simulink model "FCSMPCmono"  (R2022b)
settings: Solver=FixedStepAuto  StartTime=0.0  StopTime=5  FixedStep=Tsimu  RelTol=1e-3
undefined symbols (not defined in the file or in its folder): A, B, Izmax, Lo, Ro, Ts, Tsimu, Vdc1, Vdc2, Vgx_peak, w
libraries: spsSeriesRLCBranchLib x11, spsCurrentMeasurementLib x8, spsIGBTDiodeLib x6, slpidlib x6, simulink x4, dspstat3 x3, spsVoltageMeasurementLib x3, spsDCVoltageSourceLib x2, spsControlledVoltageSourceLib x1, spsPVArrayLib x1, spsTriangleGeneratorLib x1, spspowerguiLib x1
settings Model: Creator=hardw  LastModifiedBy=Salas Híbridas PC9
settings DebuggingCC: UnconnectedInputMsg=warning  UnconnectedOutputMsg=warning  UnconnectedLineMsg=warning
settings ModelReferenceCC: EnableRefExpFcnMdlSchedulingChecks=on
settings RTWCC: DLArmComputeVersion=19.05

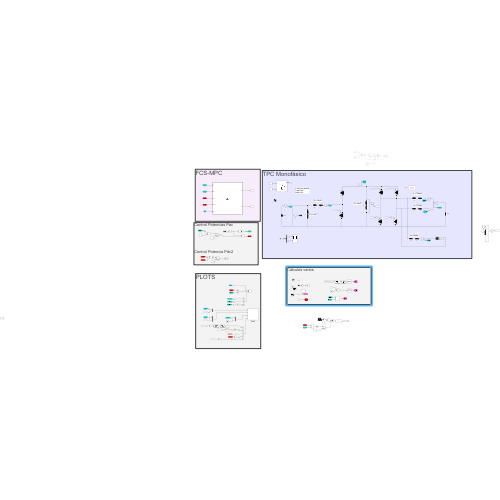
[thumbnail: Simulink's stored preview of the top-level diagram]
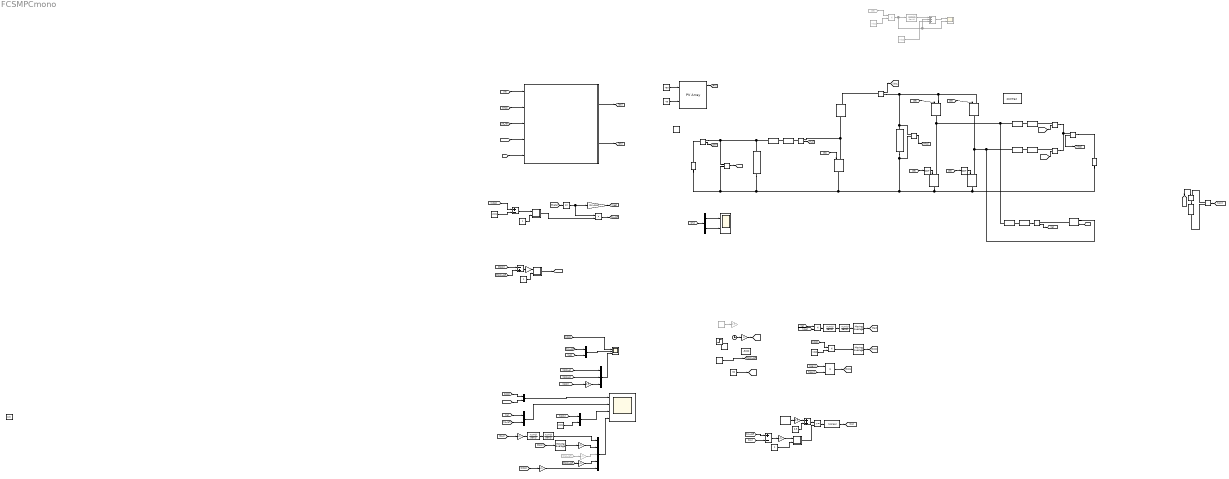
== system FCSMPCmono ==
  note: L=1mH
  note: 3 string en paralelo
      | Vmpp=42V
      | Impp=13A
  note: TPC Monofásico
  note: FCS-MPC
  note: PLOTS
  note: Control Potencias Pac
      |
      |
      |
      |
      |
      | Control Potencia Pdc2
  note: Cálculos varios
  note: C=1mF
  note: C=1mF
  note: L=10mH
  note: L=10mH
  note: L=10mH
  Bus Selector : BusSelector  OutputSignals=V_PV,I_PV
  Cast To Boolean : DataTypeConversion  OutDataTypeStr=boolean  SaturateOnIntegerOverflow=off  RndMeth=Floor
  Clock : Clock
  Constant : Constant  Value=Vdc2
  Constant1 : Constant  Value=Vdc1
  Constant10 : Constant  Value=30
  Constant11 : Constant  Value=0.5
  Constant12 : Constant  Value=750
  Constant2 : Constant  Value=45
  Constant25 : Constant  Value=0.5
  Constant3 : Constant
  Constant4 : Constant  Value=-5000
  Constant5 : Constant
  Constant6 : Constant  Commented=on  Value=Vdc1
  Constant7 : Constant  Commented=on  Value=Vdc2
  Constant8 : Constant  Value=Vdc1
  Constant9 : Constant
  Controlled Voltage Source : spsControlledVoltageSourceLib/Controlled Voltage Source  Initialize=off  Source_Type=AC  Amplitude=0  Phase=0  Frequency=0  Measurements=None
  From21 : From  Commented=on  GotoTag=Pac_ref
  From24 : From  Commented=on  GotoTag=Sa
  Gain{,1,5..6} (4 alike) : Gain  Gain=0.001
  Gain10 : Gain  Commented=on  Gain=0.5
  Gain11 : Gain  Gain=-1/Vdc1
  Gain12 : Gain  Gain=0.5
  Gain2 : Gain  Gain=0.5
  Gain3 : Gain  Gain=1e-2
  Gain32 : Gain  Gain=w
  Gain34 : Gain  Gain=Vgx_peak
  Gain4 : Gain  Commented=on  Gain=0.001
  I{1..6,8,19} (8 alike) : spsCurrentMeasurementLib/Current Measurement  PhasorSimulation=off  OutputType=Complex  PSBequivalent=0
  IGBT/Diode{1..4,27..28} (6 alike) : spsIGBTDiodeLib/IGBT//Diode  Ron=1e-3  Rs=1e5  Cs=inf  Measurements=off
  L1 : spsSeriesRLCBranchLib/Series RLC Branch  LConnTagsString=__new0  RConnTagsString=__new0  BranchType=R  Resistance=Ro  Inductance=Lo  SetiL0=off  InitialCurrent=0  Capacitance=1e-6  Setx0=off  InitialVoltage=0  Measurements=None
  L10 : spsSeriesRLCBranchLib/Series RLC Branch  LConnTagsString=__new0  RConnTagsString=__new0  BranchType=L  Resistance=Ro  Inductance=Lo  SetiL0=off  InitialCurrent=0  Capacitance=1e-6  Setx0=off  InitialVoltage=0  Measurements=None
  L13 : spsSeriesRLCBranchLib/Series RLC Branch  LConnTagsString=__new0  RConnTagsString=__new0  BranchType=RC  Resistance=Ro  Inductance=Lo  SetiL0=off  InitialCurrent=0  Capacitance=1e-3  Setx0=on  InitialVoltage=250  Measurements=None
  L18 : spsSeriesRLCBranchLib/Series RLC Branch  LConnTagsString=__new0  RConnTagsString=__new0  BranchType=RC  Resistance=Ro*0  Inductance=Lo  SetiL0=off  InitialCurrent=0  Capacitance=1e-9  Setx0=on  InitialVoltage=0  Measurements=None
  L2 : spsSeriesRLCBranchLib/Series RLC Branch  LConnTagsString=__new0  RConnTagsString=__new0  BranchType=R  Resistance=Ro  Inductance=Lo  SetiL0=off  InitialCurrent=0  Capacitance=1e-6  Setx0=off  InitialVoltage=0  Measurements=None
  L3 : spsSeriesRLCBranchLib/Series RLC Branch  LConnTagsString=__new0  RConnTagsString=__new0  BranchType=L  Resistance=Ro  Inductance=Lo  SetiL0=off  InitialCurrent=0  Capacitance=1e-6  Setx0=off  InitialVoltage=0  Measurements=None
  L4 : spsSeriesRLCBranchLib/Series RLC Branch  LConnTagsString=__new0  RConnTagsString=__new0  BranchType=L  Resistance=Ro  Inductance=Lo  SetiL0=off  InitialCurrent=0  Capacitance=1e-6  Setx0=off  InitialVoltage=0  Measurements=None
  L5 : spsSeriesRLCBranchLib/Series RLC Branch  LConnTagsString=__new0  RConnTagsString=__new0  BranchType=RC  Resistance=Ro  Inductance=Lo  SetiL0=off  InitialCurrent=0  Capacitance=1e-3  Setx0=on  InitialVoltage=100  Measurements=None
  L6 : spsSeriesRLCBranchLib/Series RLC Branch  LConnTagsString=__new0  RConnTagsString=__new0  BranchType=R  Resistance=100e-3  Inductance=Lo  SetiL0=off  InitialCurrent=0  Capacitance=1e-6  Setx0=off  InitialVoltage=0  Measurements=None
  L7 : spsSeriesRLCBranchLib/Series RLC Branch  LConnTagsString=__new0  RConnTagsString=__new0  BranchType=R  Resistance=Ro  Inductance=Lo  SetiL0=off  InitialCurrent=0  Capacitance=1e-6  Setx0=off  InitialVoltage=0  Measurements=None
  L8 : spsSeriesRLCBranchLib/Series RLC Branch  LConnTagsString=__new0  RConnTagsString=__new0  BranchType=L  Resistance=Ro  Inductance=1e-3  SetiL0=off  InitialCurrent=0  Capacitance=1e-6  Setx0=off  InitialVoltage=0  Measurements=None
  MATLAB Function2 : MATLAB Function  TreatAsAtomicUnit=on
  Moving Average : dspstat3/Moving Average  Method=Exponential weighting  ForgettingFactorPort=off  SpecifyWindowLength=on  WindowLength=4  OverlapLength=3  AllowArbitraryInputLength=off  ForgettingFactor=0.99999  SimulateUsing=Code generation
  Moving Average1 : dspstat3/Moving Average  Method=Exponential weighting  ForgettingFactorPort=off  SpecifyWindowLength=on  WindowLength=4  OverlapLength=3  AllowArbitraryInputLength=off  ForgettingFactor=0.99  SimulateUsing=Code generation
  Moving Average3 : dspstat3/Moving Average  Method=Exponential weighting  ForgettingFactorPort=off  SpecifyWindowLength=on  WindowLength=4  OverlapLength=3  AllowArbitraryInputLength=off  ForgettingFactor=0.9999  SimulateUsing=Code generation
  Mux{,1,4..5} (4 alike) : Mux  Inputs=2
  Mux2 : Mux  Inputs=5
  Mux3 : Mux  Inputs=3
  NOT1 : Logic  Operator=NOT  IconShape=distinctive  AllPortsSameDT=off  OutDataTypeStr=boolean
  NOT12 : Logic  Operator=NOT  IconShape=distinctive  AllPortsSameDT=off  OutDataTypeStr=boolean
  Notch 100Hz2 : TransferFcn  Numerator=[1 3.661 3.949e5]  Denominator=[1 628.4*2 628.4^2]
  Notch 100Hz6 : TransferFcn  Numerator=[1 3.661 3.949e5]  Denominator=[1 628.4*2 628.4^2]
  Notch 50Hz2 : TransferFcn  Numerator=[1 1.628 9.876e4]  Denominator=[1 314.3*2 314.3^2]
  Notch 50Hz4 : TransferFcn  Commented=on  Numerator=[1 1.628 9.876e4]  Denominator=[1 314.3*2 314.3^2]
  Notch 50Hz6 : TransferFcn  Numerator=[1 1.628 9.876e4]  Denominator=[1 314.3*2 314.3^2]
  PI1 : Subsystem
  PI2 : Subsystem
  PI5 : Subsystem
  PV Array : spsPVArrayLib/PV Array  Npar=3  Nser=4  PlotType=array @ 1000 W/m2 & specified temperatures  S_vec="[ 1000  500  100 ]"  Temp_C_vec="[ 45 25  ]"  ModuleName=User-defined  PlotWhenSelected=off  Pm=546  Ncell=60  Voc=50  Isc=14  Vm=42  Im=13  beta_Voc_pc=-0.36099  alpha_Isc_pc=0.102  beta_Voc=-0.18049  alpha_Isc=0.01428  IL=14.2983  I0=5.1266e-10  nI=1.3516  Rsh=65.7477  Rs=0.12608  RobustModel=off  RobustCellTemperature=313.3991  BAL=on  Tc=1e-6  Tfilter=5e-5
  Plot1 : Scope  NumInputPorts=4
  Product : Product  Commented=on
  Product{1..2,4,7} (4 alike) : Product
  Relational Operator : RelationalOperator  OutDataTypeStr=boolean  RndMeth=Simplest  InputSameDT=off
  Repeating Sequence Stair : simulink/Sources/Repeating Sequence Stair  OutValues=[750 750 750 750 750 700 700 700 700 600 600 600 600].'  tsamp=0.2  OutMin=[]  OutMax=[]  OutDataTypeStr=double  OutputDataTypeScalingMode=double  OutDataType=fixdt(0,8)  ConRadixGroup=Best Precision: Vector-wise  OutScaling=2^-12
  Repeating Sequence Stair1 : simulink/Sources/Repeating Sequence Stair  OutValues=1e3*[0 0 0 -5 -5 -5 -10 -10 0 0 5 5 5 5].'  tsamp=0.2  OutMin=[]  OutMax=[]  OutDataTypeStr=double  OutputDataTypeScalingMode=double  OutDataType=fixdt(0,8)  ConRadixGroup=Best Precision: Vector-wise  OutScaling=2^-12
  Repeating Sequence Stair2 : simulink/Sources/Repeating Sequence Stair  OutValues=1e3*[0 -5 -10].'  tsamp=1.5  OutMin=[]  OutMax=[]  OutDataTypeStr=double  OutputDataTypeScalingMode=double  OutDataType=fixdt(0,8)  ConRadixGroup=Best Precision: Vector-wise  OutScaling=2^-12
  Repeating Sequence Stair4 : simulink/Sources/Repeating Sequence Stair  Commented=on  OutValues=-1e3*[10 10 10 5 5 0 0 -10 -10 -10 -10].'  tsamp=0.2  OutMin=[]  OutMax=[]  OutDataTypeStr=double  OutputDataTypeScalingMode=double  OutDataType=fixdt(0,8)  ConRadixGroup=Best Precision: Vector-wise  OutScaling=2^-12
  Scope1 : Scope  Commented=on  NumInputPorts=2
  Scope5 : Scope  NumInputPorts=3
  Scope6 : Scope  NumInputPorts=2
  Sin : Trigonometry
  Step : Step  Time=1.5  After=-5000  SampleTime=0
  Sum of Elements2 : Sum  Inputs=-+
  Sum of Elements3 : Sum  Commented=on  Inputs=-++
  Sum of Elements4 : Sum  Inputs=+-
  Sum of Elements5 : Sum  Inputs=+-
  Sum of Elements6 : Sum
  Triangle Generator : spsTriangleGeneratorLib/Triangle Generator  Freq=25e3  Phase=90  Ts=0
  V1 : spsVoltageMeasurementLib/Voltage Measurement  PhasorSimulation=off  OutputType=Complex  PSBequivalent=0
  V2 : spsVoltageMeasurementLib/Voltage Measurement  PhasorSimulation=off  OutputType=Complex  PSBequivalent=0
  V4 : spsVoltageMeasurementLib/Voltage Measurement  PhasorSimulation=off  OutputType=Complex  PSBequivalent=0
  VDC1 : spsDCVoltageSourceLib/DC Voltage Source  Amplitude=Vdc2  Measurements=None
  VDC2 : spsDCVoltageSourceLib/DC Voltage Source  Amplitude=150  Measurements=None
  powergui : spspowerguiLib/powergui  Priority=1  SimulationMode=Discrete  SampleTime=Tsimu  frequency=60  Iterations=50  frequencyindice=0  Pbase=100e6  ErrMax=1e-4  UnitsV=kV  UnitsW=MW  buscounter=0  FunctionMessages=off  echomessages=off  EnableUseOfTLC=off  CurrentSourceSwitches=off  DisableSnubberDevices=off  DisableRonSwitches=off  DisableVfSwitches=off  DisplayEquations=off  AutomaticDiscreteSolvers=off  SolverType=Tustin/Backward Euler (TBE)  Interpol=off  ExternalGateDelay=off  methode=off  Ts=100  x0status=blocks  SPID=off  SwTol=0  HookPort=off  NonlinearTolerance=1e-4  nMaxIteration=100  ContinueOnMaxIteration=off  RestoreLinks=warning  ResistiveCurrentMeasurement=off  Frange=[0:2:500]  Ylog=off  Xlog=on  ShowGrid=off  save=off  variable=ZData  structure=Iza  ZoomFFT=on  StartTime=0.3  cycles=1  DisplayStyle=1  fundamental=50  FreqAxis=off  MaxFrequency=25000  frequencyindicesteady=1  RmsSteady=1  display=off
  wires:
  NOT12/1 -> IGBT/Diode28/1
  [Sa] -> IGBT/Diode27/1
  NOT1/1 -> IGBT/Diode2/1
  [Sb] -> IGBT/Diode1/1
  I3/1 -> [Ia]
  [Ia] -> Product1/1
  [Vga] -> Controlled Voltage Source/1
  [Vga] -> Product1/2
  I19/1 -> [Idc2]
  Sin/1 -> Gain34/1, Product4/1
  Clock/1 -> Gain32/1
  Gain32/1 -> [theta]
  [theta] -> Sin/1
  Gain34/1 -> [Vga]
  [Vga] -> MATLAB Function2/5(Vag)
  Product4/1 -> [Ia_ref]
  [Ia_ref] -> MATLAB Function2/3(ia_ref)
  [Idc2_ref] -> MATLAB Function2/4(idc2_ref)
  [Idc2] -> MATLAB Function2/2(idc2)
  [Ia] -> MATLAB Function2/1(ia)
  MATLAB Function2/1(Sa) -> [Sa]  "Sa"
  MATLAB Function2/2(Sb) -> [Sb]  "Sb"
  [Idc2] -> Mux/1  "Idc2"
  [Idc2_ref] -> Mux/2  "Idc2*"
  Mux/1 -> Plot1/1
  Mux1/1 -> Plot1/2
  [Ia] -> Mux1/1  "Ia"
  [Ia_ref] -> Mux1/2  "Ia*"
  [Idc2] -> Product7/1
  Constant/1 -> Product7/2
  Notch 50Hz6/1 -> Mux2/1  "Pac"
  Gain1/1 -> Mux2/2  "Pdc2"
  Mux2/1 -> Plot1/4
  Moving Average/1 -> [Pac]
  Moving Average1/1 -> [Pdc2]
  Product7/1 -> Moving Average1/1
  I1/1 -> [Idc1]
  Moving Average3/1 -> Gain1/1  "Pdc2"
  Constant3/1 -> PI5/2(en)  "Iuc"
  PI1/1(o) -> [Idc2_ref]  "izc_ref"
  Constant5/1 -> PI1/2(en)  "Iuc"
  Sum of Elements2/1 -> Gain3/1
  Gain3/1 -> PI1/1(e)
  [Pdc2] -> Sum of Elements2/1  "Pdc"
  [Pdc2_ref] -> Sum of Elements2/2
  [Pdc2] -> Moving Average3/1  "Pdc2"
  From21/1 -> Gain4/1
  [Pdc2_ref] -> Gain5/1
  Gain4/1 -> Mux2/3  "Pac*"
  Gain5/1 -> Mux2/4  "Pdc2*"
  [Idc1] -> Scope5/1  "Idc1"
  PI5/1(o) -> Product4/2  "izc_ref"
  V4/1 -> [Vcm]
  I8/1 -> [Icm]  "Icm"
  Notch 100Hz6/1 -> Notch 50Hz6/1
  [Pac] -> Gain/1  "Pac"
  Gain/1 -> Notch 100Hz6/1  "Pac"
  [Pdc1] -> Gain6/1
  Gain6/1 -> Mux2/5  "Pdc1"
  I5/1 -> [Idc2_a]
  I6/1 -> [Idc2_b]
  [Sa] -> NOT12/1
  [Sb] -> NOT1/1
  Notch 100Hz2/1 -> Notch 50Hz2/1
  Product1/1 -> Notch 100Hz2/1
  Notch 50Hz2/1 -> Moving Average/1  "Pac"
  [Idc2_a] -> Mux3/1  "Idc2_a"
  [Idc2_b] -> Mux3/2  "Idc2_b"
  Mux3/1 -> Scope5/3
  From24/1 -> Product/1
  Constant6/1 -> Product/2
  Product/1 -> Scope1/2, Sum of Elements3/2, Notch 50Hz4/1
  Notch 50Hz4/1 -> Sum of Elements3/1  "Pdc1"
  Sum of Elements3/1 -> Scope1/1
  Constant7/1 -> Sum of Elements3/3
  Gain2/1 -> Mux3/3  "Idc2/2"
  V2/1 -> [Vdc1]
  [Idc2] -> Gain2/1  "Idc2"
  [Vdc1] -> Sum of Elements4/1  "Pdc"
  Constant8/1 -> Sum of Elements4/2  "Iuc"
  Sum of Elements4/1 -> PI5/1(e)
  Repeating Sequence Stair2/1 -> [Pdc2_ref]
  Sum of Elements5/1 -> Gain11/1
  Gain11/1 -> PI2/1(e)
  Constant9/1 -> PI2/2(en)  "Iuc"
  Triangle Generator/1 -> Gain12/1
  Gain12/1 -> Sum of Elements6/1
  Constant11/1 -> Sum of Elements6/2
  Sum of Elements6/1 -> Relational Operator/1  "Carrier"
  Relational Operator/1 -> Cast To Boolean/1
  Cast To Boolean/1 -> [S1]  "S"
  PI2/1(o) -> Relational Operator/2  "d"
  I2/1 -> [IL1]
  [IL1] -> Sum of Elements5/2  "I"
  [S1] -> IGBT/Diode4/1
  [IL1_ref] -> Sum of Elements5/1  "I*"
  Constant2/1 -> PV Array/2
  Constant12/1 -> PV Array/1
  PV Array/1 -> [PV]
  [PV] -> Bus Selector/1
  Bus Selector/1 -> Scope6/1  "<V_PV>"
  Bus Selector/2 -> Scope6/2  "<I_PV>"
  Repeating Sequence Stair4/1 -> Gain10/1
  Constant10/1 -> [IL1_ref]  "I*"
  Product2/1 -> [Pdc1]
  [IL1] -> Mux5/2  "I"
  [IL1_ref] -> Mux5/1  "I*"
  Mux5/1 -> Scope5/2
  [Vdc1] -> Mux4/1  "Vdc"
  Constant1/1 -> Mux4/2  "Vdc*"
  Mux4/1 -> Plot1/3
  V1/1 -> [Vpan]
  I4/1 -> [Ipan]
  [Ipan] -> Product2/1  "I"
  [Vpan] -> Product2/2  "I"
  connections:
  L2/LConn1 -- L3/RConn1
  L1/LConn1 -- L4/RConn1
  IGBT/Diode28/LConn1 -- L4/LConn1 -- L10/LConn1 -- IGBT/Diode27/RConn1
  IGBT/Diode27/LConn1 -- I1/RConn1 -- V2/LConn1 -- L13/LConn1 -- IGBT/Diode1/LConn1
  L7/LConn1 -- L10/RConn1
  L7/RConn1 -- I3/LConn1
  Controlled Voltage Source/RConn1 -- I3/RConn1
  I19/LConn1 -- VDC1/RConn1
  I8/LConn1 -- L18/LConn1
  IGBT/Diode2/LConn1 -- Controlled Voltage Source/LConn1 -- L3/LConn1 -- IGBT/Diode1/RConn1
  L13/RConn1 -- V2/LConn2 -- VDC2/LConn1 -- V1/LConn2 -- L5/RConn1 -- IGBT/Diode4/RConn1 -- VDC1/LConn1 -- IGBT/Diode2/RConn1 -- IGBT/Diode28/RConn1
  I5/RConn1 -- L1/RConn1
  I5/LConn1 -- I6/LConn1 -- I19/RConn1
  I6/RConn1 -- L2/RConn1
  L6/LConn1 -- L8/RConn1
  L5/LConn1 -- V1/LConn1 -- I4/RConn1 -- L8/LConn1
  IGBT/Diode3/LConn1 -- I1/LConn1
  IGBT/Diode4/LConn1 -- I2/RConn1 -- IGBT/Diode3/RConn1
  I2/LConn1 -- L6/RConn1
  V4/LConn2 -- L18/RConn1
  V4/LConn1 -- I8/RConn1
  I4/LConn1 -- VDC2/RConn1

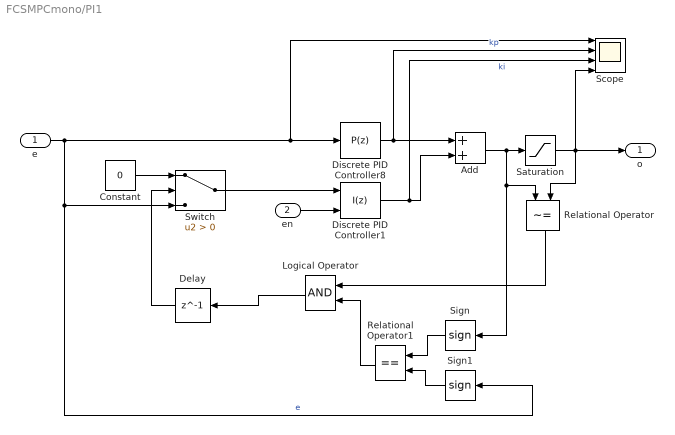
== system FCSMPCmono/PI1 ==
  e : Inport
  en : Inport  Port=2
  Add : Sum
  Constant : Constant  Value=0
  Delay : Delay  DelayLength=1  InitialCondition=0
  Discrete PID Controller1 : slpidlib/PID Controller  Controller=I  Form=Parallel  TimeDomain=Discrete-time  UseExternalTs=off  SampleTime=-1  IntegratorMethod=Trapezoidal  FilterMethod=Forward Euler  ControllerParametersSource=internal  P=0.17337190810745  I=10  UseKiTs=off  D=0  N=100  UseFilter=on  TunerSelectOption=Transfer Function Based (PID Tuner App)  InitialConditionSource=internal  InitialConditionForIntegrator=0  InitialConditionForFilter=0  DifferentiatorICPrevScaledInput=0  ExternalReset=rising  TrackingMode=off  Kt=1  LimitOutput=off  SatLimitsSource=internal  UpperSaturationLimit=Izmax  LowerSaturationLimit=-Izmax  LinearizeAsGain=off  AntiWindupMode=clamping  Kb=1  LimitIntegrator=off  UpperIntegratorSaturationLimit=inf  LowerIntegratorSaturationLimit=-inf  POutMin=[]  POutMax=[]  IOutMin=[]  IOutMax=[]  DOutMin=[]  DOutMax=[]  NOutMin=[]  NOutMax=[]  SumOutMin=[]  SumOutMax=[]  SaturationOutMin=[]  SaturationOutMax=[]  PParamMin=[]  PParamMax=[]  IParamMin=[]  IParamMax=[]  DParamMin=[]  DParamMax=[]  NParamMin=[]  NParamMax=[]  KbParamMin=[]  KbParamMax=[]  KtParamMin=[]  KtParamMax=[]  KbOutMin=[]  KbOutMax=[]  KtOutMin=[]  KtOutMax=[]  IntegratorOutMin=[]  IntegratorOutMax=[]  FilterOutMin=[]  FilterOutMax=[]  SumI1OutMin=[]  SumI1OutMax=[]  SumI2OutMin=[]  SumI2OutMax=[]  SumI3OutMin=[]  SumI3OutMax=[]  SumI4OutMin=[]  SumI4OutMax=[]  SumDOutMin=[]  SumDOutMax=[]  DifferentiatorOutMin=[]  DifferentiatorOutMax=[]  FilterDiffOutCoefMin=[]  FilterDiffOutCoefMax=[]  ReciprocalOutMin=[]  ReciprocalOutMax=[]  SumDenOutMin=[]  SumDenOutMax=[]  SumNumOutMin=[]  SumNumOutMax=[]  DivideOutMin=[]  DivideOutMax=[]  UdiffTsProdOutMin=[]  UdiffTsProdOutMax=[]  NTsProdOutMin=[]  NTsProdOutMax=[]  UintegralTsProdOutMin=[]  UintegralTsProdOutMax=[]  UngainTsProdOutMin=[]  UngainTsProdOutMax=[]  ClampingZeroOutDataTypeStr=Inherit: Inherit via back propagation  ClampingZeroOutMin=[]  ClampingZeroOutMax=[]  FilterDenConstantOutDataTypeStr=Inherit: Inherit via back propagation  FilterDenConstantOutMin=[]  FilterDenConstantOutMax=[]  PCopyOutDataTypeStr=Inherit: Inherit via back propagation  PCopyOutMin=[]  PCopyOutMax=[]  NCopyOutDataTypeStr=Inherit: Inherit via back propagation  NCopyOutMin=[]  NCopyOutMax=[]  IntegratorContinuousStateAttributes=''  IntegratorStateMustResolveToSignalObject=off  IntegratorRTWStateStorageClass=Auto  FilterContinuousStateAttributes=''  FilterStateMustResolveToSignalObject=off  FilterRTWStateStorageClass=Auto  ParallelPVariant=Disabled  IdealPVariant=Disabled  IVariant=InternalParameters  DVariant=Disabled  IntegratorVariant=Discrete  SatVariant=Disabled  AWVariant=Passthrough  PCopyVariant=Disabled  TRVariant=Disabled  FdbkBlocksVariant=Forward  IdealPFdbkVariant=Disabled  SatFdbkVariant=Disabled  DerivativeFilterVariant=Disabled  NVariant=Disabled  NCopyVariant=Disabled_SignalSpec  FilterICVariant=Disabled  IntegratorICVariant=InternalICs  ExternalResetVariant=ExternalReset  TRSumVariant=Passthrough  SumFdbkVariant=Disabled  SumVariant=Passthrough_I  TsampFilterVariant=InternalTs  TsampNgainVariant=Passthrough  TsampIntegralVariant=Passthrough  ExternalSaturationOutDataTypeStr=Inherit: Same as second input
  Discrete PID Controller8 : slpidlib/PID Controller  Controller=P  Form=Parallel  TimeDomain=Discrete-time  UseExternalTs=off  SampleTime=-1  IntegratorMethod=Trapezoidal  FilterMethod=Forward Euler  ControllerParametersSource=internal  P=0.01  I=4.00000740741931  UseKiTs=off  D=0  N=100  UseFilter=on  TunerSelectOption=Frequency Response Based  InitialConditionSource=internal  InitialConditionForIntegrator=0  InitialConditionForFilter=0  DifferentiatorICPrevScaledInput=0  ExternalReset=none  TrackingMode=off  Kt=1  LimitOutput=off  SatLimitsSource=internal  UpperSaturationLimit=Izmax  LowerSaturationLimit=-Izmax  LinearizeAsGain=off  AntiWindupMode=clamping  Kb=1  LimitIntegrator=off  UpperIntegratorSaturationLimit=inf  LowerIntegratorSaturationLimit=-inf  POutMin=[]  POutMax=[]  IOutMin=[]  IOutMax=[]  DOutMin=[]  DOutMax=[]  NOutMin=[]  NOutMax=[]  SumOutMin=[]  SumOutMax=[]  SaturationOutMin=[]  SaturationOutMax=[]  PParamMin=[]  PParamMax=[]  IParamMin=[]  IParamMax=[]  DParamMin=[]  DParamMax=[]  NParamMin=[]  NParamMax=[]  KbParamMin=[]  KbParamMax=[]  KtParamMin=[]  KtParamMax=[]  KbOutMin=[]  KbOutMax=[]  KtOutMin=[]  KtOutMax=[]  IntegratorOutMin=[]  IntegratorOutMax=[]  FilterOutMin=[]  FilterOutMax=[]  SumI1OutMin=[]  SumI1OutMax=[]  SumI2OutMin=[]  SumI2OutMax=[]  SumI3OutMin=[]  SumI3OutMax=[]  SumI4OutMin=[]  SumI4OutMax=[]  SumDOutMin=[]  SumDOutMax=[]  DifferentiatorOutMin=[]  DifferentiatorOutMax=[]  FilterDiffOutCoefMin=[]  FilterDiffOutCoefMax=[]  ReciprocalOutMin=[]  ReciprocalOutMax=[]  SumDenOutMin=[]  SumDenOutMax=[]  SumNumOutMin=[]  SumNumOutMax=[]  DivideOutMin=[]  DivideOutMax=[]  UdiffTsProdOutMin=[]  UdiffTsProdOutMax=[]  NTsProdOutMin=[]  NTsProdOutMax=[]  UintegralTsProdOutMin=[]  UintegralTsProdOutMax=[]  UngainTsProdOutMin=[]  UngainTsProdOutMax=[]  ClampingZeroOutDataTypeStr=Inherit: Inherit via back propagation  ClampingZeroOutMin=[]  ClampingZeroOutMax=[]  FilterDenConstantOutDataTypeStr=Inherit: Inherit via back propagation  FilterDenConstantOutMin=[]  FilterDenConstantOutMax=[]  PCopyOutDataTypeStr=Inherit: Inherit via back propagation  PCopyOutMin=[]  PCopyOutMax=[]  NCopyOutDataTypeStr=Inherit: Inherit via back propagation  NCopyOutMin=[]  NCopyOutMax=[]  IntegratorContinuousStateAttributes=''  IntegratorStateMustResolveToSignalObject=off  IntegratorRTWStateStorageClass=Auto  FilterContinuousStateAttributes=''  FilterStateMustResolveToSignalObject=off  FilterRTWStateStorageClass=Auto  ParallelPVariant=InternalParameters  IdealPVariant=Disabled  IVariant=Disabled  DVariant=Disabled  IntegratorVariant=Disabled  SatVariant=Disabled  AWVariant=Disabled  PCopyVariant=Disabled  TRVariant=Disabled  FdbkBlocksVariant=Forward  IdealPFdbkVariant=Disabled  SatFdbkVariant=Disabled  DerivativeFilterVariant=Disabled  NVariant=Disabled  NCopyVariant=Disabled_SignalSpec  FilterICVariant=Disabled  IntegratorICVariant=Disabled  ExternalResetVariant=Disabled  TRSumVariant=Passthrough  SumFdbkVariant=Disabled  SumVariant=Passthrough_P  TsampFilterVariant=InternalTs  TsampNgainVariant=Passthrough  TsampIntegralVariant=Disabled_SignalSpec  ExternalSaturationOutDataTypeStr=Inherit: Same as second input
  Logical Operator : Logic  AllPortsSameDT=off  OutDataTypeStr=boolean
  Relational Operator : RelationalOperator  Operator=~=  OutDataTypeStr=boolean  InputSameDT=off
  Relational Operator1 : RelationalOperator  Operator===  OutDataTypeStr=boolean  InputSameDT=off
  Saturation : Saturate  UpperLimit=80  LowerLimit=-80
  Scope : Scope  NumInputPorts=4
  Sign : Signum
  Sign1 : Signum
  Switch : Switch  Criteria=u2 > Threshold  SaturateOnIntegerOverflow=off  InputSameDT=off
  o : Outport  VectorParamsAs1DForOutWhenUnconnected=off
  wires:
  en/1 -> Discrete PID Controller1/2
  Delay/1 -> Switch/2
  Relational Operator1/1 -> Logical Operator/2
  Relational Operator/1 -> Logical Operator/1
  Sign1/1 -> Relational Operator1/2
  Sign/1 -> Relational Operator1/1
  Constant/1 -> Switch/1
  Logical Operator/1 -> Delay/1
  Switch/1 -> Discrete PID Controller1/1
  Add/1 -> Saturation/1, Sign/1, Relational Operator/1
  Discrete PID Controller1/1 -> Add/2, Scope/3  "ki"
  Discrete PID Controller8/1 -> Add/1, Scope/2  "kp"
  Saturation/1 -> o/1, Relational Operator/2, Scope/4
  e/1 -> Sign1/1, Switch/3, Discrete PID Controller8/1, Scope/1  "e"

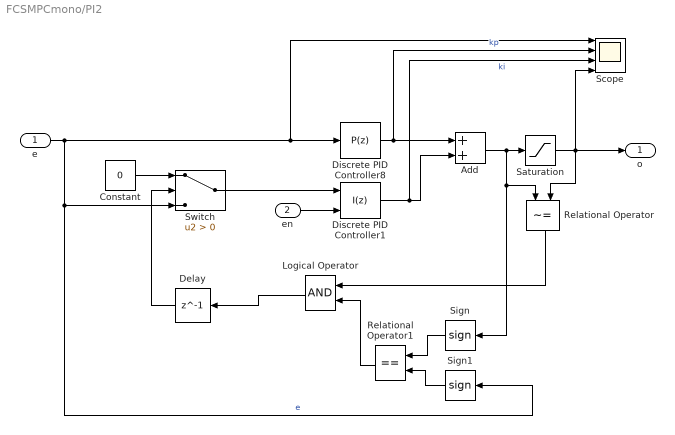
== system FCSMPCmono/PI2 ==
  e : Inport
  en : Inport  Port=2
  Add : Sum
  Constant : Constant  Value=0
  Delay : Delay  DelayLength=1  InitialCondition=0
  Discrete PID Controller1 : slpidlib/PID Controller  Controller=I  Form=Parallel  TimeDomain=Discrete-time  UseExternalTs=off  SampleTime=-1  IntegratorMethod=Trapezoidal  FilterMethod=Forward Euler  ControllerParametersSource=internal  P=0.17337190810745  I=100  UseKiTs=off  D=0  N=100  UseFilter=on  TunerSelectOption=Transfer Function Based (PID Tuner App)  InitialConditionSource=internal  InitialConditionForIntegrator=0.38  InitialConditionForFilter=0  DifferentiatorICPrevScaledInput=0  ExternalReset=rising  TrackingMode=off  Kt=1  LimitOutput=off  SatLimitsSource=internal  UpperSaturationLimit=Izmax  LowerSaturationLimit=-Izmax  LinearizeAsGain=off  AntiWindupMode=clamping  Kb=1  LimitIntegrator=off  UpperIntegratorSaturationLimit=inf  LowerIntegratorSaturationLimit=-inf  POutMin=[]  POutMax=[]  IOutMin=[]  IOutMax=[]  DOutMin=[]  DOutMax=[]  NOutMin=[]  NOutMax=[]  SumOutMin=[]  SumOutMax=[]  SaturationOutMin=[]  SaturationOutMax=[]  PParamMin=[]  PParamMax=[]  IParamMin=[]  IParamMax=[]  DParamMin=[]  DParamMax=[]  NParamMin=[]  NParamMax=[]  KbParamMin=[]  KbParamMax=[]  KtParamMin=[]  KtParamMax=[]  KbOutMin=[]  KbOutMax=[]  KtOutMin=[]  KtOutMax=[]  IntegratorOutMin=[]  IntegratorOutMax=[]  FilterOutMin=[]  FilterOutMax=[]  SumI1OutMin=[]  SumI1OutMax=[]  SumI2OutMin=[]  SumI2OutMax=[]  SumI3OutMin=[]  SumI3OutMax=[]  SumI4OutMin=[]  SumI4OutMax=[]  SumDOutMin=[]  SumDOutMax=[]  DifferentiatorOutMin=[]  DifferentiatorOutMax=[]  FilterDiffOutCoefMin=[]  FilterDiffOutCoefMax=[]  ReciprocalOutMin=[]  ReciprocalOutMax=[]  SumDenOutMin=[]  SumDenOutMax=[]  SumNumOutMin=[]  SumNumOutMax=[]  DivideOutMin=[]  DivideOutMax=[]  UdiffTsProdOutMin=[]  UdiffTsProdOutMax=[]  NTsProdOutMin=[]  NTsProdOutMax=[]  UintegralTsProdOutMin=[]  UintegralTsProdOutMax=[]  UngainTsProdOutMin=[]  UngainTsProdOutMax=[]  ClampingZeroOutDataTypeStr=Inherit: Inherit via back propagation  ClampingZeroOutMin=[]  ClampingZeroOutMax=[]  FilterDenConstantOutDataTypeStr=Inherit: Inherit via back propagation  FilterDenConstantOutMin=[]  FilterDenConstantOutMax=[]  PCopyOutDataTypeStr=Inherit: Inherit via back propagation  PCopyOutMin=[]  PCopyOutMax=[]  NCopyOutDataTypeStr=Inherit: Inherit via back propagation  NCopyOutMin=[]  NCopyOutMax=[]  IntegratorContinuousStateAttributes=''  IntegratorStateMustResolveToSignalObject=off  IntegratorRTWStateStorageClass=Auto  FilterContinuousStateAttributes=''  FilterStateMustResolveToSignalObject=off  FilterRTWStateStorageClass=Auto  ParallelPVariant=Disabled  IdealPVariant=Disabled  IVariant=InternalParameters  DVariant=Disabled  IntegratorVariant=Discrete  SatVariant=Disabled  AWVariant=Passthrough  PCopyVariant=Disabled  TRVariant=Disabled  FdbkBlocksVariant=Forward  IdealPFdbkVariant=Disabled  SatFdbkVariant=Disabled  DerivativeFilterVariant=Disabled  NVariant=Disabled  NCopyVariant=Disabled_SignalSpec  FilterICVariant=Disabled  IntegratorICVariant=InternalICs  ExternalResetVariant=ExternalReset  TRSumVariant=Passthrough  SumFdbkVariant=Disabled  SumVariant=Passthrough_I  TsampFilterVariant=InternalTs  TsampNgainVariant=Passthrough  TsampIntegralVariant=Passthrough  ExternalSaturationOutDataTypeStr=Inherit: Same as second input
  Discrete PID Controller8 : slpidlib/PID Controller  Controller=P  Form=Parallel  TimeDomain=Discrete-time  UseExternalTs=off  SampleTime=-1  IntegratorMethod=Trapezoidal  FilterMethod=Forward Euler  ControllerParametersSource=internal  P=10  I=4.00000740741931  UseKiTs=off  D=0  N=100  UseFilter=on  TunerSelectOption=Frequency Response Based  InitialConditionSource=internal  InitialConditionForIntegrator=0  InitialConditionForFilter=0  DifferentiatorICPrevScaledInput=0  ExternalReset=none  TrackingMode=off  Kt=1  LimitOutput=off  SatLimitsSource=internal  UpperSaturationLimit=Izmax  LowerSaturationLimit=-Izmax  LinearizeAsGain=off  AntiWindupMode=clamping  Kb=1  LimitIntegrator=off  UpperIntegratorSaturationLimit=inf  LowerIntegratorSaturationLimit=-inf  POutMin=[]  POutMax=[]  IOutMin=[]  IOutMax=[]  DOutMin=[]  DOutMax=[]  NOutMin=[]  NOutMax=[]  SumOutMin=[]  SumOutMax=[]  SaturationOutMin=[]  SaturationOutMax=[]  PParamMin=[]  PParamMax=[]  IParamMin=[]  IParamMax=[]  DParamMin=[]  DParamMax=[]  NParamMin=[]  NParamMax=[]  KbParamMin=[]  KbParamMax=[]  KtParamMin=[]  KtParamMax=[]  KbOutMin=[]  KbOutMax=[]  KtOutMin=[]  KtOutMax=[]  IntegratorOutMin=[]  IntegratorOutMax=[]  FilterOutMin=[]  FilterOutMax=[]  SumI1OutMin=[]  SumI1OutMax=[]  SumI2OutMin=[]  SumI2OutMax=[]  SumI3OutMin=[]  SumI3OutMax=[]  SumI4OutMin=[]  SumI4OutMax=[]  SumDOutMin=[]  SumDOutMax=[]  DifferentiatorOutMin=[]  DifferentiatorOutMax=[]  FilterDiffOutCoefMin=[]  FilterDiffOutCoefMax=[]  ReciprocalOutMin=[]  ReciprocalOutMax=[]  SumDenOutMin=[]  SumDenOutMax=[]  SumNumOutMin=[]  SumNumOutMax=[]  DivideOutMin=[]  DivideOutMax=[]  UdiffTsProdOutMin=[]  UdiffTsProdOutMax=[]  NTsProdOutMin=[]  NTsProdOutMax=[]  UintegralTsProdOutMin=[]  UintegralTsProdOutMax=[]  UngainTsProdOutMin=[]  UngainTsProdOutMax=[]  ClampingZeroOutDataTypeStr=Inherit: Inherit via back propagation  ClampingZeroOutMin=[]  ClampingZeroOutMax=[]  FilterDenConstantOutDataTypeStr=Inherit: Inherit via back propagation  FilterDenConstantOutMin=[]  FilterDenConstantOutMax=[]  PCopyOutDataTypeStr=Inherit: Inherit via back propagation  PCopyOutMin=[]  PCopyOutMax=[]  NCopyOutDataTypeStr=Inherit: Inherit via back propagation  NCopyOutMin=[]  NCopyOutMax=[]  IntegratorContinuousStateAttributes=''  IntegratorStateMustResolveToSignalObject=off  IntegratorRTWStateStorageClass=Auto  FilterContinuousStateAttributes=''  FilterStateMustResolveToSignalObject=off  FilterRTWStateStorageClass=Auto  ParallelPVariant=InternalParameters  IdealPVariant=Disabled  IVariant=Disabled  DVariant=Disabled  IntegratorVariant=Disabled  SatVariant=Disabled  AWVariant=Disabled  PCopyVariant=Disabled  TRVariant=Disabled  FdbkBlocksVariant=Forward  IdealPFdbkVariant=Disabled  SatFdbkVariant=Disabled  DerivativeFilterVariant=Disabled  NVariant=Disabled  NCopyVariant=Disabled_SignalSpec  FilterICVariant=Disabled  IntegratorICVariant=Disabled  ExternalResetVariant=Disabled  TRSumVariant=Passthrough  SumFdbkVariant=Disabled  SumVariant=Passthrough_P  TsampFilterVariant=InternalTs  TsampNgainVariant=Passthrough  TsampIntegralVariant=Disabled_SignalSpec  ExternalSaturationOutDataTypeStr=Inherit: Same as second input
  Logical Operator : Logic  AllPortsSameDT=off  OutDataTypeStr=boolean
  Relational Operator : RelationalOperator  Operator=~=  OutDataTypeStr=boolean  InputSameDT=off
  Relational Operator1 : RelationalOperator  Operator===  OutDataTypeStr=boolean  InputSameDT=off
  Saturation : Saturate  UpperLimit=1  LowerLimit=0
  Scope : Scope  NumInputPorts=4
  Sign : Signum
  Sign1 : Signum
  Switch : Switch  Criteria=u2 > Threshold  SaturateOnIntegerOverflow=off  InputSameDT=off
  o : Outport  VectorParamsAs1DForOutWhenUnconnected=off
  wires:
  en/1 -> Discrete PID Controller1/2
  Delay/1 -> Switch/2
  Relational Operator1/1 -> Logical Operator/2
  Relational Operator/1 -> Logical Operator/1
  Sign1/1 -> Relational Operator1/2
  Sign/1 -> Relational Operator1/1
  Constant/1 -> Switch/1
  Logical Operator/1 -> Delay/1
  Switch/1 -> Discrete PID Controller1/1
  Add/1 -> Saturation/1, Sign/1, Relational Operator/1
  Discrete PID Controller1/1 -> Add/2, Scope/3  "ki"
  Discrete PID Controller8/1 -> Add/1, Scope/2  "kp"
  Saturation/1 -> o/1, Relational Operator/2, Scope/4
  e/1 -> Sign1/1, Switch/3, Discrete PID Controller8/1, Scope/1  "e"

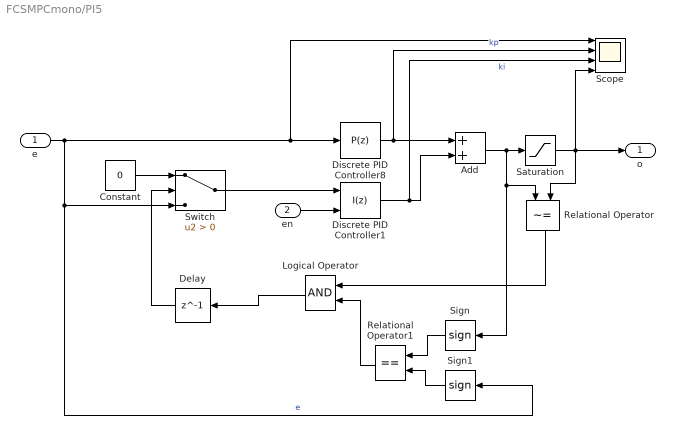
== system FCSMPCmono/PI5 ==
  e : Inport
  en : Inport  Port=2
  Add : Sum
  Constant : Constant  Value=0
  Delay : Delay  DelayLength=1  InitialCondition=0
  Discrete PID Controller1 : slpidlib/PID Controller  Controller=I  Form=Parallel  TimeDomain=Discrete-time  UseExternalTs=off  SampleTime=-1  IntegratorMethod=Trapezoidal  FilterMethod=Forward Euler  ControllerParametersSource=internal  P=0.17337190810745  I=10  UseKiTs=off  D=0  N=100  UseFilter=on  TunerSelectOption=Transfer Function Based (PID Tuner App)  InitialConditionSource=internal  InitialConditionForIntegrator=0  InitialConditionForFilter=0  DifferentiatorICPrevScaledInput=0  ExternalReset=rising  TrackingMode=off  Kt=1  LimitOutput=off  SatLimitsSource=internal  UpperSaturationLimit=Izmax  LowerSaturationLimit=-Izmax  LinearizeAsGain=off  AntiWindupMode=clamping  Kb=1  LimitIntegrator=off  UpperIntegratorSaturationLimit=inf  LowerIntegratorSaturationLimit=-inf  POutMin=[]  POutMax=[]  IOutMin=[]  IOutMax=[]  DOutMin=[]  DOutMax=[]  NOutMin=[]  NOutMax=[]  SumOutMin=[]  SumOutMax=[]  SaturationOutMin=[]  SaturationOutMax=[]  PParamMin=[]  PParamMax=[]  IParamMin=[]  IParamMax=[]  DParamMin=[]  DParamMax=[]  NParamMin=[]  NParamMax=[]  KbParamMin=[]  KbParamMax=[]  KtParamMin=[]  KtParamMax=[]  KbOutMin=[]  KbOutMax=[]  KtOutMin=[]  KtOutMax=[]  IntegratorOutMin=[]  IntegratorOutMax=[]  FilterOutMin=[]  FilterOutMax=[]  SumI1OutMin=[]  SumI1OutMax=[]  SumI2OutMin=[]  SumI2OutMax=[]  SumI3OutMin=[]  SumI3OutMax=[]  SumI4OutMin=[]  SumI4OutMax=[]  SumDOutMin=[]  SumDOutMax=[]  DifferentiatorOutMin=[]  DifferentiatorOutMax=[]  FilterDiffOutCoefMin=[]  FilterDiffOutCoefMax=[]  ReciprocalOutMin=[]  ReciprocalOutMax=[]  SumDenOutMin=[]  SumDenOutMax=[]  SumNumOutMin=[]  SumNumOutMax=[]  DivideOutMin=[]  DivideOutMax=[]  UdiffTsProdOutMin=[]  UdiffTsProdOutMax=[]  NTsProdOutMin=[]  NTsProdOutMax=[]  UintegralTsProdOutMin=[]  UintegralTsProdOutMax=[]  UngainTsProdOutMin=[]  UngainTsProdOutMax=[]  ClampingZeroOutDataTypeStr=Inherit: Inherit via back propagation  ClampingZeroOutMin=[]  ClampingZeroOutMax=[]  FilterDenConstantOutDataTypeStr=Inherit: Inherit via back propagation  FilterDenConstantOutMin=[]  FilterDenConstantOutMax=[]  PCopyOutDataTypeStr=Inherit: Inherit via back propagation  PCopyOutMin=[]  PCopyOutMax=[]  NCopyOutDataTypeStr=Inherit: Inherit via back propagation  NCopyOutMin=[]  NCopyOutMax=[]  IntegratorContinuousStateAttributes=''  IntegratorStateMustResolveToSignalObject=off  IntegratorRTWStateStorageClass=Auto  FilterContinuousStateAttributes=''  FilterStateMustResolveToSignalObject=off  FilterRTWStateStorageClass=Auto  ParallelPVariant=Disabled  IdealPVariant=Disabled  IVariant=InternalParameters  DVariant=Disabled  IntegratorVariant=Discrete  SatVariant=Disabled  AWVariant=Passthrough  PCopyVariant=Disabled  TRVariant=Disabled  FdbkBlocksVariant=Forward  IdealPFdbkVariant=Disabled  SatFdbkVariant=Disabled  DerivativeFilterVariant=Disabled  NVariant=Disabled  NCopyVariant=Disabled_SignalSpec  FilterICVariant=Disabled  IntegratorICVariant=InternalICs  ExternalResetVariant=ExternalReset  TRSumVariant=Passthrough  SumFdbkVariant=Disabled  SumVariant=Passthrough_I  TsampFilterVariant=InternalTs  TsampNgainVariant=Passthrough  TsampIntegralVariant=Passthrough  ExternalSaturationOutDataTypeStr=Inherit: Same as second input
  Discrete PID Controller8 : slpidlib/PID Controller  Controller=P  Form=Parallel  TimeDomain=Discrete-time  UseExternalTs=off  SampleTime=-1  IntegratorMethod=Trapezoidal  FilterMethod=Forward Euler  ControllerParametersSource=internal  P=0.5  I=4.00000740741931  UseKiTs=off  D=0  N=100  UseFilter=on  TunerSelectOption=Frequency Response Based  InitialConditionSource=internal  InitialConditionForIntegrator=0  InitialConditionForFilter=0  DifferentiatorICPrevScaledInput=0  ExternalReset=none  TrackingMode=off  Kt=1  LimitOutput=off  SatLimitsSource=internal  UpperSaturationLimit=Izmax  LowerSaturationLimit=-Izmax  LinearizeAsGain=off  AntiWindupMode=clamping  Kb=1  LimitIntegrator=off  UpperIntegratorSaturationLimit=inf  LowerIntegratorSaturationLimit=-inf  POutMin=[]  POutMax=[]  IOutMin=[]  IOutMax=[]  DOutMin=[]  DOutMax=[]  NOutMin=[]  NOutMax=[]  SumOutMin=[]  SumOutMax=[]  SaturationOutMin=[]  SaturationOutMax=[]  PParamMin=[]  PParamMax=[]  IParamMin=[]  IParamMax=[]  DParamMin=[]  DParamMax=[]  NParamMin=[]  NParamMax=[]  KbParamMin=[]  KbParamMax=[]  KtParamMin=[]  KtParamMax=[]  KbOutMin=[]  KbOutMax=[]  KtOutMin=[]  KtOutMax=[]  IntegratorOutMin=[]  IntegratorOutMax=[]  FilterOutMin=[]  FilterOutMax=[]  SumI1OutMin=[]  SumI1OutMax=[]  SumI2OutMin=[]  SumI2OutMax=[]  SumI3OutMin=[]  SumI3OutMax=[]  SumI4OutMin=[]  SumI4OutMax=[]  SumDOutMin=[]  SumDOutMax=[]  DifferentiatorOutMin=[]  DifferentiatorOutMax=[]  FilterDiffOutCoefMin=[]  FilterDiffOutCoefMax=[]  ReciprocalOutMin=[]  ReciprocalOutMax=[]  SumDenOutMin=[]  SumDenOutMax=[]  SumNumOutMin=[]  SumNumOutMax=[]  DivideOutMin=[]  DivideOutMax=[]  UdiffTsProdOutMin=[]  UdiffTsProdOutMax=[]  NTsProdOutMin=[]  NTsProdOutMax=[]  UintegralTsProdOutMin=[]  UintegralTsProdOutMax=[]  UngainTsProdOutMin=[]  UngainTsProdOutMax=[]  ClampingZeroOutDataTypeStr=Inherit: Inherit via back propagation  ClampingZeroOutMin=[]  ClampingZeroOutMax=[]  FilterDenConstantOutDataTypeStr=Inherit: Inherit via back propagation  FilterDenConstantOutMin=[]  FilterDenConstantOutMax=[]  PCopyOutDataTypeStr=Inherit: Inherit via back propagation  PCopyOutMin=[]  PCopyOutMax=[]  NCopyOutDataTypeStr=Inherit: Inherit via back propagation  NCopyOutMin=[]  NCopyOutMax=[]  IntegratorContinuousStateAttributes=''  IntegratorStateMustResolveToSignalObject=off  IntegratorRTWStateStorageClass=Auto  FilterContinuousStateAttributes=''  FilterStateMustResolveToSignalObject=off  FilterRTWStateStorageClass=Auto  ParallelPVariant=InternalParameters  IdealPVariant=Disabled  IVariant=Disabled  DVariant=Disabled  IntegratorVariant=Disabled  SatVariant=Disabled  AWVariant=Disabled  PCopyVariant=Disabled  TRVariant=Disabled  FdbkBlocksVariant=Forward  IdealPFdbkVariant=Disabled  SatFdbkVariant=Disabled  DerivativeFilterVariant=Disabled  NVariant=Disabled  NCopyVariant=Disabled_SignalSpec  FilterICVariant=Disabled  IntegratorICVariant=Disabled  ExternalResetVariant=Disabled  TRSumVariant=Passthrough  SumFdbkVariant=Disabled  SumVariant=Passthrough_P  TsampFilterVariant=InternalTs  TsampNgainVariant=Passthrough  TsampIntegralVariant=Disabled_SignalSpec  ExternalSaturationOutDataTypeStr=Inherit: Same as second input
  Logical Operator : Logic  AllPortsSameDT=off  OutDataTypeStr=boolean
  Relational Operator : RelationalOperator  Operator=~=  OutDataTypeStr=boolean  InputSameDT=off
  Relational Operator1 : RelationalOperator  Operator===  OutDataTypeStr=boolean  InputSameDT=off
  Saturation : Saturate  UpperLimit=110  LowerLimit=-110
  Scope : Scope  NumInputPorts=4
  Sign : Signum
  Sign1 : Signum
  Switch : Switch  Criteria=u2 > Threshold  SaturateOnIntegerOverflow=off  InputSameDT=off
  o : Outport  VectorParamsAs1DForOutWhenUnconnected=off
  wires:
  e/1 -> Scope/1, Discrete PID Controller8/1, Switch/3, Sign1/1  "e"
  Saturation/1 -> Scope/4, Relational Operator/2, o/1
  Discrete PID Controller8/1 -> Scope/2, Add/1  "kp"
  Discrete PID Controller1/1 -> Scope/3, Add/2  "ki"
  Add/1 -> Relational Operator/1, Sign/1, Saturation/1
  Switch/1 -> Discrete PID Controller1/1
  Logical Operator/1 -> Delay/1
  Constant/1 -> Switch/1
  Sign/1 -> Relational Operator1/1
  Sign1/1 -> Relational Operator1/2
  Relational Operator/1 -> Logical Operator/1
  Relational Operator1/1 -> Logical Operator/2
  Delay/1 -> Switch/2
  en/1 -> Discrete PID Controller1/2

== matlab function FCSMPCmono/MATLAB Function2 ==
  settings: updateMethod=DISCRETE  sampleTime=Ts
  data: ia input; Sa output; idc2 input; ia_ref input; idc2_ref input; Sb output; Vag input; Vdc2 parameter; A parameter; B parameter; Ts parameter; Vdc1 parameter; Lo parameter
function [Sa,Sb]= FCSMPC(ia,idc2,ia_ref,idc2_ref,Vag,Vdc2,A, B, Ts, Vdc1,Lo)
persistent Sold
if isempty(Sold) 
    Sold=[0;0];
end
lambda=0.01;
d=1/Lo*[-Vag;2*Vdc2];
x=[ia;idc2];
x_ref=[ia_ref;idc2_ref];

FCS=[0 0;...
     0 1;...
     1 0;...
     1 1 ]*Vdc1;
Jmin=10000;
Q=[1 0;...
   0 100];
S=[0;1];
for i = 1:4
    %as=FCS(i,:)'
    xk1=(eye(2)+Ts*A)*x+Ts*B*FCS(i,:)'+Ts*d;
    J=(xk1-x_ref)'*Q*(xk1-x_ref)+lambda*norm(FCS(i,:)'-Sold);
    if J<Jmin
        Jmin=J;
        S=FCS(i,:)'/Vdc1;
    end

end
Sa=S(1,1);
Sb=S(2,1);
Sold=S;

end
